simulink model "elastic_joint_param_estim"  (R2024b)
settings: Solver=FixedStepAuto  StartTime=0.0  StopTime=20  FixedStep=0.001  RelTol=1e-3
undefined symbols (not defined in the file or in its folder): DiscIntNeverNeededParam, National_Instruments, PCI, sens, Ts
libraries: sldrtlib x1, simulink x1
settings Model: SimulationMode=external  ExtModeTrigDuration=50001  ExtModeTrigDurationFloating=50001  Creator=perondavid  LastModifiedBy=bassanienr
settings DataIOCC: LoggingToFile=on
settings OptimizationCC: ReuseModelBlockBuffer=off
settings HardwareCC: ProdBitPerLong=64  ProdHWDeviceType=Intel->x86-64 (Linux 64)
settings RTWCC: Description=Simulink Desktop Real-Time  SystemTargetFile=sldrt.tlc  TemplateMakefile=sldrt.tmf  RTWCompilerOptimization=on  GPUComputeCapability=3.5
settings CodeAppCC: MaxIdLength=95
settings SimulinkDesktopRealTimeCC: TargetLibSuffix=_sldrt.a  TargetPreCompLibLocation=C:\Program Files\MATLAB\R2024b\toolbox\sldrt\lib\win64  ParMdlRefBuildCompliant=on

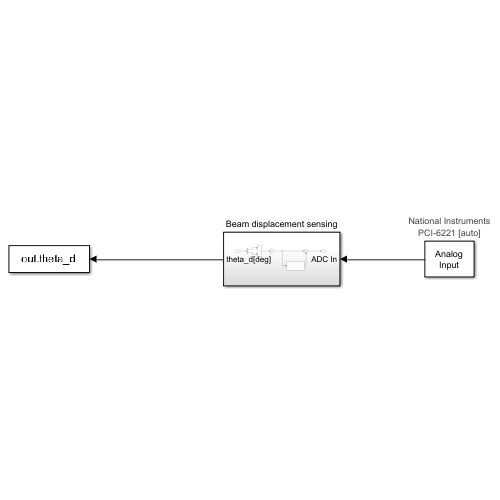
[thumbnail: Simulink's stored preview of the top-level diagram]
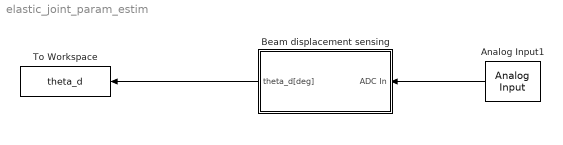
== system elastic_joint_param_estim ==
  Analog Input1 : sldrtlib/Analog Input  SampleTime=-1  MaxMissedTicks=10  ShowMissedTicks=off  YieldWhenWaiting=off  DrvName=National_Instruments/PCI-6221  DrvAddress=4294967295  DrvOptions=[0 0 0 2 0]  Channels=[3, 4]  RangeMode=1  VoltRange=2  DataType=1
      settings: AttributesFormatString=National Instruments\nPCI-6221 [auto]
  Beam displacement sensing : Subsystem
  To Workspace : ToWorkspace  VariableName=theta_d  SaveFormat=Structure With Time  SampleTime=Ts
  wires:
  Beam displacement sensing/1(theta_d[deg]) -> To Workspace/1
  Analog Input1/1 -> Beam displacement sensing/1(ADC In)

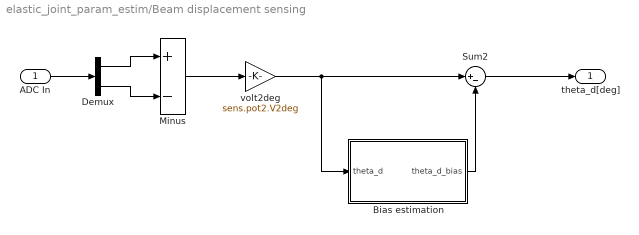
== system elastic_joint_param_estim/Beam displacement sensing ==
  ADC In : Inport
  " Bias estimation" : Subsystem
  Demux : Demux  Outputs=2
  Minus : Sum  Inputs=+-
  Sum2 : Sum  Inputs=|+-
  volt2deg : Gain  Gain=sens.pot2.V2deg
  theta_d[deg] : Outport
  wires:
  volt2deg/1 -> " Bias estimation"/1(theta_d), Sum2/1
  Sum2/1 -> theta_d[deg]/1
  " Bias estimation"/1(theta_d_bias) -> Sum2/2
  Minus/1 -> volt2deg/1
  Demux/2 -> Minus/2
  ADC In/1 -> Demux/1
  Demux/1 -> Minus/1

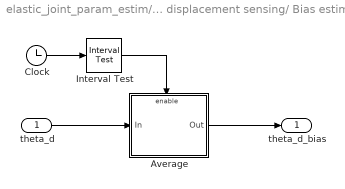
== system elastic_joint_param_estim/Beam displacement sensing/ Bias estimation ==
  theta_d : Inport
  Average : Subsystem
  Clock : Clock
  Interval Test : simulink/Logic and Bit Operations/Interval Test  IntervalClosedRight=on  uplimit=0.7  IntervalClosedLeft=on  lowlimit=0.2  OutDataTypeStr=boolean
  theta_d_bias : Outport
  wires:
  Clock/1 -> Interval Test/1
  theta_d/1 -> Average/1(In)
  Interval Test/1 -> Average/Enable
  Average/1(Out) -> theta_d_bias/1

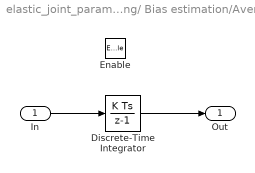
== system elastic_joint_param_estim/Beam displacement sensing/ Bias estimation/Average ==
  In : Inport
  Enable : EnablePort
  Discrete-Time Integrator : DiscreteIntegrator  SampleTime=Ts  ICPrevOutput=DiscIntNeverNeededParam  ICPrevScaledInput=DiscIntNeverNeededParam
  Out : Outport
  wires:
  In/1 -> Discrete-Time Integrator/1
  Discrete-Time Integrator/1 -> Out/1
